simulink model "CopyModel"  (R2019b)
settings: Solver=VariableStepAuto  StartTime=0.0  StopTime=10.0  RelTol=1e-3
values from neighbouring files (symbols this model uses):
  etcModeCmd = 0    [F28379D_benchTest_CPU1.sldd]
  etcModes : value not decoded    [F28379D_benchTest_CPU1.sldd]
  etcSubModeCmd = 0    [F28379D_benchTest_CPU1.sldd]
  etcSubModes : value not decoded    [F28379D_benchTest_CPU1.sldd]
  motorControlMode = 0    [F28379D_benchTest_CPU1.sldd]
  motorPosGainI = 0.0    [F28379D_benchTest_CPU1.sldd]
  motorPosGainP = 2000.0    [F28379D_benchTest_CPU1.sldd]
  motorVelGainFeedback = 200.0    [F28379D_benchTest_CPU1.sldd]
  motorVelGainI = 2000.0    [F28379D_benchTest_CPU1.sldd]
  motorVelGainP = 200.0    [F28379D_benchTest_CPU1.sldd]
  throttlePosInputMode = 0    [F28379D_benchTest_CPU1.sldd]
  throttlePosInputModes : value not decoded    [F28379D_benchTest_CPU1.sldd]
undefined symbols (not defined in the file or in its folder): motor1PWM, motor2PWM, motorPosCommand_deg
libraries: simulink x30, c280xlib x10, canmsglib x9, FunctionCallDivider x6, hdlsllib x1
settings Model: Creator=zacha  LastModifiedBy=Nick

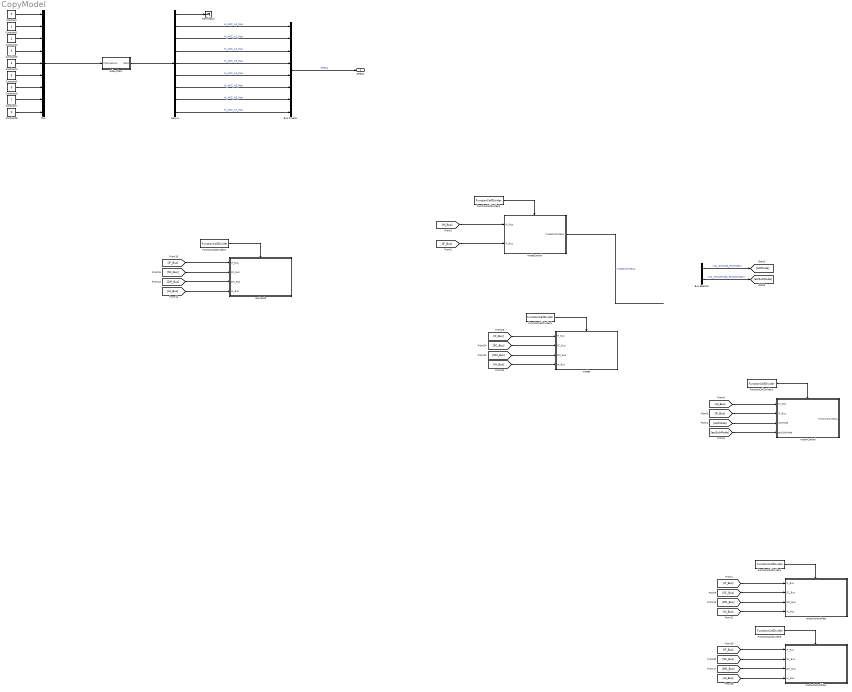
== system CopyModel ==
  Bus Creator : BusCreator  Inputs=8
  Bus Selector : BusSelector  OutputSignals=modeControlBus.SC_etcMode_etcModes,modeControlBus.SC_etcSubMode_etcSubModes
  Constant : Constant  Value=0
  Constant1 : Constant
  Constant2 : Constant  Value=2
  Constant3 : Constant  Value=3
  Constant4 : Constant  Value=4
  Constant5 : Constant  Value=5
  Constant6 : Constant  Value=6
  Constant7 : Constant  Value=7
  Constant8 : Constant  Value=0
  Demux : Demux  Outputs=9
  FunctionCallDivider1 : FunctionCallDivider/Algroithms/FunctionCallDivider  counts=1
  FunctionCallDivider2 : FunctionCallDivider/Algroithms/FunctionCallDivider  counts=10
  FunctionCallDivider3 : FunctionCallDivider/Algroithms/FunctionCallDivider  counts=10
  FunctionCallDivider4 : FunctionCallDivider/Algroithms/FunctionCallDivider  counts=1
  FunctionCallDivider5 : FunctionCallDivider/Algroithms/FunctionCallDivider  counts=100
  FunctionCallDivider6 : FunctionCallDivider/Algroithms/FunctionCallDivider  counts=10
  Mux : Mux  Inputs=9
  Subsystem : Subsystem
  Terminator : Terminator
  modeControl : Subsystem  TreatAsAtomicUnit=on
  modes : Subsystem  TreatAsAtomicUnit=on
  motorControl : Subsystem  TreatAsAtomicUnit=on
  motorControlFast : Subsystem  TreatAsAtomicUnit=on
  motorControlSlow : Subsystem  TreatAsAtomicUnit=on
  rawInputs : Subsystem  TreatAsAtomicUnit=on
  SPIBus : Outport
  wires:
  Demux/5 -> Bus Creator/4  "HI_ADC_A3_Raw"
  Bus Creator/1 -> SPIBus/1  "SPIBus"
  Constant4/1 -> Mux/5
  Mux/1 -> Subsystem/1(ChannelNum)
  Demux/7 -> Bus Creator/6  "HI_ADC_A5_Raw"
  Demux/4 -> Bus Creator/3  "HI_ADC_A2_Raw"
  Demux/2 -> Bus Creator/1  "HI_ADC_A0_Raw"
  Constant1/1 -> Mux/2
  Demux/3 -> Bus Creator/2  "HI_ADC_A1_Raw"
  Demux/8 -> Bus Creator/7  "HI_ADC_A6_Raw"
  Demux/9 -> Bus Creator/8  "HI_ADC_A7_Raw"
  Constant7/1 -> Mux/8
  Constant2/1 -> Mux/3
  Constant8/1 -> Mux/9
  Constant5/1 -> Mux/6
  Demux/6 -> Bus Creator/5  "HI_ADC_A4_Raw"
  Subsystem/1(Data) -> Demux/1
  Constant3/1 -> Mux/4
  Demux/1 -> Terminator/1
  Constant6/1 -> Mux/7
  Constant/1 -> Mux/1
  FunctionCallDivider3/1 -> rawInputs/Trigger
  [SC_Bus] -> rawInputs/2(SC_Bus)
  [IF_Bus] -> rawInputs/1(IF_Bus)
  [HI_Bus] -> rawInputs/4(HI_Bus)
  [DM_Bus] -> rawInputs/3(DM_Bus)
  [HI_Bus] -> modeControl/1(HI_Bus)
  Bus Selector/2 -> [etcSubMode]  "<SC_etcSubMode_etcSubModes>"
  modeControl/1(modeControlBus) -> ?  "modeControlBus"
  FunctionCallDivider2/1 -> modeControl/Trigger
  Bus Selector/1 -> [etcMode]  "<SC_etcMode_etcModes>"
  ? -> Bus Selector/1  "SC_Bus"
  [IF_Bus] -> modeControl/2(IF_Bus)
  [SC_Bus] -> modes/2(SC_Bus)
  FunctionCallDivider5/1 -> modes/Trigger
  [DM_Bus] -> modes/3(DM_Bus)
  [HI_Bus] -> modes/4(HI_Bus)
  [IF_Bus] -> modes/1(IF_Bus)
  FunctionCallDivider1/1 -> motorControl/Trigger
  [IF_Bus] -> motorControl/2(IF_Bus)
  [etcSubMode] -> motorControl/4(etcSubMode)
  [HI_Bus] -> motorControl/1(HI_Bus)
  [etcMode] -> motorControl/3(etcMode)
  FunctionCallDivider4/1 -> motorControlFast/Trigger
  [IF_Bus] -> motorControlSlow/1(IF_Bus)
  [DM_Bus] -> motorControlFast/3(DM_Bus)
  [SC_Bus] -> motorControlSlow/2(SC_Bus)
  [DM_Bus] -> motorControlSlow/3(DM_Bus)
  [HI_Bus] -> motorControlSlow/4(HI_Bus)
  FunctionCallDivider6/1 -> motorControlSlow/Trigger
  [HI_Bus] -> motorControlFast/4(HI_Bus)
  [IF_Bus] -> motorControlFast/1(IF_Bus)
  [SC_Bus] -> motorControlFast/2(SC_Bus)

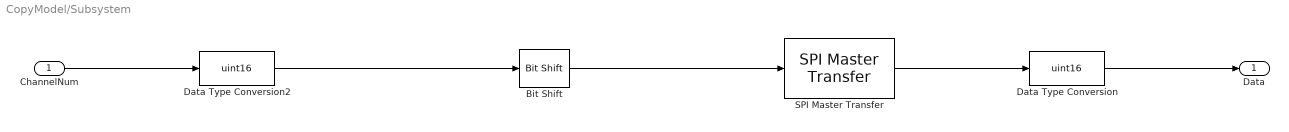
== system CopyModel/Subsystem ==
  ChannelNum : Inport
  Bit Shift : hdlsllib/Logic and Bit Operations/Bit Shift  mode=Shift Left Logical  N=11
      settings: SourceProductName=Simulink
  Data Type Conversion : DataTypeConversion  OutDataTypeStr=uint16
  Data Type Conversion2 : DataTypeConversion  OutDataTypeStr=uint16
  SPI Master Transfer : c280xlib/SPI Master Transfer  SPISelect=SPI_B  ClockPolarity=Falling_edge  ClockPhase=No_delay  SPIModule=uint32(0)  Mode=Master  BusSpeed=uint32(1000000)  FirstBitToTransfer=Most significant bit (MSB)  ClockMode=0  BlockFunction=Transfer  EnableRegisterAddress=on  RegisterAddress=0  OutputDataType=int8  OutputDataLength=1  DataBits=16  UseCustomSSPin=Explicit GPIO calls  ActiveLowSSPin=Active low  Pin=66
      settings: SourceProductName=Embedded Coder Support Package for Texas Instruments C2000 Processors  SourceProductBaseCode=TIC2000
  Data : Outport
  wires:
  ChannelNum/1 -> Data Type Conversion2/1
  Data Type Conversion/1 -> Data/1
  SPI Master Transfer/1 -> Data Type Conversion/1
  Data Type Conversion2/1 -> Bit Shift/1
  Bit Shift/1 -> SPI Master Transfer/1

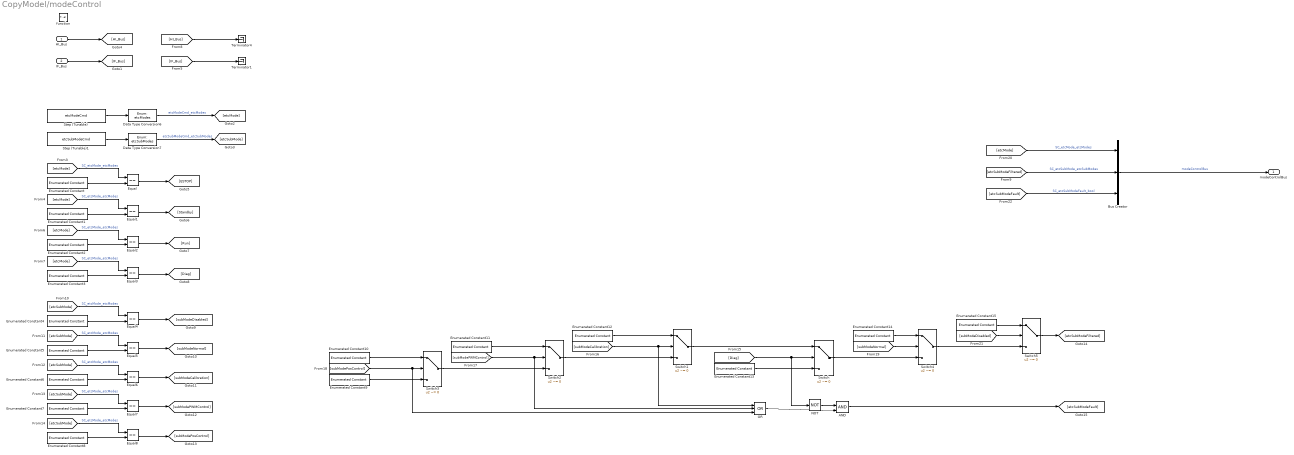
== system CopyModel/modeControl ==
  HI_Bus : Inport
  IF_Bus : Inport  Port=2
  function : TriggerPort  TriggerType=function-call  VariantControl=Variant
  AND : Logic  IconShape=distinctive  AllPortsSameDT=off  OutDataTypeStr=boolean
  Bus Creator : BusCreator  Inputs=3
  Data Type Conversion6 : DataTypeConversion  OutDataTypeStr=Enum: etcModes
  Data Type Conversion7 : DataTypeConversion  OutDataTypeStr=Enum: etcSubModes
  Enumerated Constant : simulink/Sources/Enumerated Constant  OutDataTypeStr=Enum: etcModes  Value=etcModes.ESTOP  SampleTime=inf
      settings: SourceProductName=Simulink
  Enumerated Constant1 : simulink/Sources/Enumerated Constant  OutDataTypeStr=Enum: etcModes  Value=etcModes.Standby  SampleTime=inf
      settings: SourceProductName=Simulink
  Enumerated Constant10 : simulink/Sources/Enumerated Constant  OutDataTypeStr=Enum: etcSubModes  Value=etcSubModes.PositionControl  SampleTime=inf
      settings: SourceProductName=Simulink
  Enumerated Constant11 : simulink/Sources/Enumerated Constant  OutDataTypeStr=Enum: etcSubModes  Value=etcSubModes.PWMControl  SampleTime=inf
      settings: SourceProductName=Simulink
  Enumerated Constant12 : simulink/Sources/Enumerated Constant  OutDataTypeStr=Enum: etcSubModes  Value=etcSubModes.Calibration  SampleTime=inf
      settings: SourceProductName=Simulink
  Enumerated Constant{4,9,13,15} (4 alike) : simulink/Sources/Enumerated Constant  OutDataTypeStr=Enum: etcSubModes  Value=etcSubModes.Disabled  SampleTime=inf
      settings: SourceProductName=Simulink
  Enumerated Constant14 : simulink/Sources/Enumerated Constant  OutDataTypeStr=Enum: etcSubModes  Value=etcSubModes.Normal  SampleTime=inf
      settings: SourceProductName=Simulink
  Enumerated Constant2 : simulink/Sources/Enumerated Constant  OutDataTypeStr=Enum: etcModes  Value=etcModes.Run  SampleTime=inf
      settings: SourceProductName=Simulink
  Enumerated Constant3 : simulink/Sources/Enumerated Constant  OutDataTypeStr=Enum: etcModes  Value=etcModes.Diag  SampleTime=inf
      settings: SourceProductName=Simulink
  Enumerated Constant5 : simulink/Sources/Enumerated Constant  OutDataTypeStr=Enum: etcSubModes  Value=etcSubModes.Normal  SampleTime=inf
      settings: SourceProductName=Simulink
  Enumerated Constant6 : simulink/Sources/Enumerated Constant  OutDataTypeStr=Enum: etcSubModes  Value=etcSubModes.Calibration  SampleTime=inf
      settings: SourceProductName=Simulink
  Enumerated Constant7 : simulink/Sources/Enumerated Constant  OutDataTypeStr=Enum: etcSubModes  Value=etcSubModes.PWMControl  SampleTime=inf
      settings: SourceProductName=Simulink
  Enumerated Constant8 : simulink/Sources/Enumerated Constant  OutDataTypeStr=Enum: etcSubModes  Value=etcSubModes.PositionControl  SampleTime=inf
      settings: SourceProductName=Simulink
  Equal{,1..8} (9 alike) : RelationalOperator  Operator===  OutDataTypeStr=boolean  RndMeth=Simplest
  NOT : Logic  Operator=NOT  IconShape=distinctive  AllPortsSameDT=off  OutDataTypeStr=boolean
  OR : Logic  Operator=OR  Inputs=3  IconShape=distinctive  AllPortsSameDT=off  OutDataTypeStr=boolean
  Step (Tunable) : Constant  Value=etcModeCmd  VectorParams1D=off  SampleTime=-1
  Step (Tunable)1 : Constant  Value=etcSubModeCmd  VectorParams1D=off  SampleTime=-1
  Switch{,1..5} (6 alike) : Switch  Criteria=u2 ~= 0
  Terminator1 : Terminator
  Terminator4 : Terminator
  modeControlBus : Outport
  wires:
  IF_Bus/1 -> [IF_Bus]
  [HI_Bus] -> Terminator4/1
  HI_Bus/1 -> [HI_Bus]
  [IF_Bus] -> Terminator1/1
  Bus Creator/1 -> modeControlBus/1  "modeControlBus"
  [etcMode] -> Bus Creator/1  "SC_etcMode_etcModes"
  [etcMode] -> Equal/1  "SC_etcMode_etcModes"
  Enumerated Constant/1 -> Equal/2
  Equal/1 -> [ESTOP]
  Equal1/1 -> [Standby]
  [etcMode] -> Equal1/1  "SC_etcMode_etcModes"
  Enumerated Constant1/1 -> Equal1/2
  Equal2/1 -> [Run]
  Enumerated Constant2/1 -> Equal2/2
  [etcMode] -> Equal2/1  "SC_etcMode_etcModes"
  Enumerated Constant3/1 -> Equal3/2
  [etcMode] -> Equal3/1  "SC_etcMode_etcModes"
  Equal3/1 -> [Diag]
  [etcSubModeFiltered] -> Bus Creator/2  "SC_etcSubMode_etcSubModes"
  Equal4/1 -> [subModeDisabled]
  [etcSubMode] -> Equal4/1  "SC_etcMode_etcModes"
  Enumerated Constant4/1 -> Equal4/2
  Enumerated Constant5/1 -> Equal5/2
  Equal5/1 -> [subModeNormal]
  [etcSubMode] -> Equal5/1  "SC_etcMode_etcModes"
  Enumerated Constant6/1 -> Equal6/2
  Equal6/1 -> [subModeCalibration]
  [etcSubMode] -> Equal6/1  "SC_etcMode_etcModes"
  Enumerated Constant7/1 -> Equal7/2
  Equal7/1 -> [subModePWMControl]
  [etcSubMode] -> Equal7/1  "SC_etcMode_etcModes"
  Enumerated Constant8/1 -> Equal8/2
  Equal8/1 -> [subModePosControl]
  [etcSubMode] -> Equal8/1  "SC_etcMode_etcModes"
  [Diag] -> NOT/1, Switch/2
  Switch1/1 -> Switch/1
  [subModeCalibration] -> OR/1, Switch1/2
  [subModePWMControl] -> OR/2, Switch2/2
  Switch2/1 -> Switch1/3
  [subModePosControl] -> OR/3, Switch3/2
  Switch3/1 -> Switch2/3
  Enumerated Constant9/1 -> Switch3/3
  Enumerated Constant10/1 -> Switch3/1
  Enumerated Constant11/1 -> Switch2/1
  Enumerated Constant12/1 -> Switch1/1
  Enumerated Constant13/1 -> Switch/3
  Switch/1 -> Switch4/3
  [subModeNormal] -> Switch4/2
  Enumerated Constant14/1 -> Switch4/1
  Enumerated Constant15/1 -> Switch5/1
  Switch4/1 -> Switch5/3
  [subModeDisabled] -> Switch5/2
  Switch5/1 -> [etcSubModeFiltered]
  OR/1 -> AND/2
  AND/1 -> [etcSubModeFault]
  [etcSubModeFault] -> Bus Creator/3  "SC_etcSubModeFault_bool"
  NOT/1 -> AND/1
  Step (Tunable)1/1 -> Data Type Conversion7/1
  Data Type Conversion7/1 -> [etcSubMode]  "etcSubModeCmd_etcSubModes"
  Step (Tunable)/1 -> Data Type Conversion6/1
  Data Type Conversion6/1 -> [etcMode]  "etcModeCmd_etcModes"

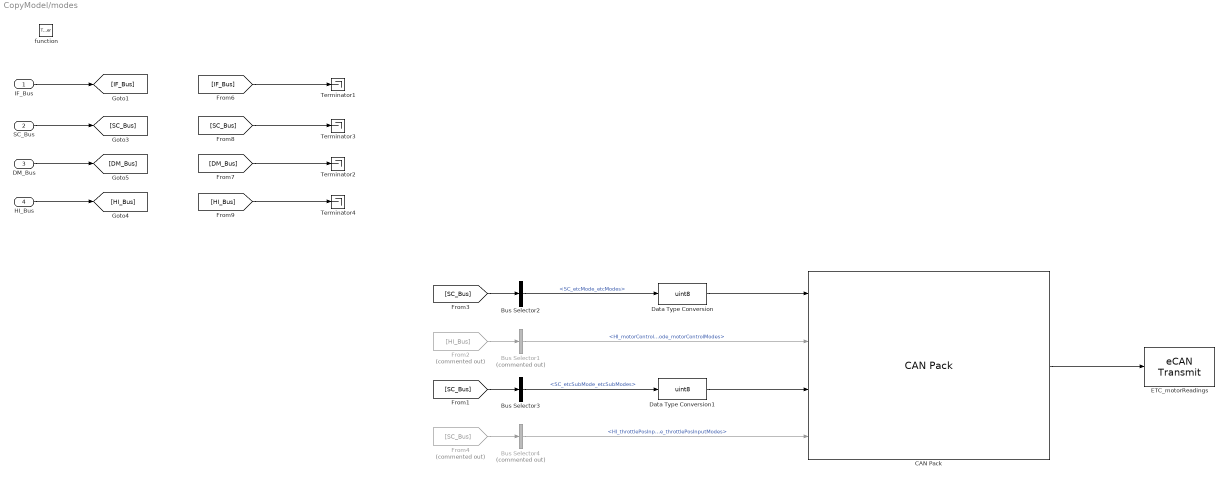
== system CopyModel/modes ==
  IF_Bus : Inport
  SC_Bus : Inport  Port=2
  DM_Bus : Inport  Port=3
  HI_Bus : Inport  Port=4
  function : TriggerPort  TriggerType=function-call  VariantControl=Variant
  Bus Selector1 : BusSelector  Commented=on  OutputSignals=VectorBoxBus.HI_motorControlMode_motorControlModes
  Bus Selector2 : BusSelector  OutputSignals=modeControlBus.SC_etcMode_etcModes
  Bus Selector3 : BusSelector  OutputSignals=modeControlBus.SC_etcSubMode_etcSubModes
  Bus Selector4 : BusSelector  Commented=on  OutputSignals=VectorBoxBus.HI_throttlePosInputMode_throttlePosInputModes
  CAN Pack : canmsglib/CAN Pack  CANdbFile=C:\Git\ETC-Development\DBCs\F28377S_etc_benchTest.dbc  MsgList=ETC_modes  MsgName=ETC_modes  MsgIDType=Standard (11-bit identifier)  MsgIdentifier=1000  MsgLength=4  Remote=off  ApplyMinMax=off  BusOutput=off  SignalInfo={'ETC_mode','0','8','LE','unsigned','Standard','0','1','0','0','255';'ETC_motorControlMode','16','8','LE','unsigned','Standard','0','1','0','0','255';'ETC_subMode','8','8','LE','unsigned','Standard','0','1','0','0','255';'ETC_throttlePosInputMode','24','8','LE','unsigned','Standard','0','1','0','0','255'}
      settings: SourceProductName=Vehicle Network Toolbox  SourceProductBaseCode=VN  DataFormat=CANdb specified signals
  Data Type Conversion : DataTypeConversion  OutDataTypeStr=uint8
  Data Type Conversion1 : DataTypeConversion  OutDataTypeStr=uint8
  ETC_motorReadings : c280xlib/eCAN Transmit  chipFamily=C280x  useModule=eCAN_A  mailboxNo=13  messageID=0  messageType=Standard (11-bit identifier)  enableBlockingMode=off  postInterrupt=off  interruptLine=0
      settings: SourceProductName=Embedded Coder Support Package for Texas Instruments C2000 Processors  SourceProductBaseCode=TIC2000
  From2 : From  Commented=on  GotoTag=HI_Bus
  From4 : From  Commented=on  GotoTag=SC_Bus
  Terminator{1..4} (4 alike) : Terminator
  wires:
  From4/1 -> Bus Selector4/1
  Bus Selector4/1 -> CAN Pack/4  "<HI_throttlePosInputMode_throttlePosInputModes>"
  [SC_Bus] -> Bus Selector3/1
  Bus Selector3/1 -> Data Type Conversion1/1  "<SC_etcSubMode_etcSubModes>"
  IF_Bus/1 -> [IF_Bus]
  [HI_Bus] -> Terminator4/1
  HI_Bus/1 -> [HI_Bus]
  SC_Bus/1 -> [SC_Bus]
  DM_Bus/1 -> [DM_Bus]
  [SC_Bus] -> Terminator3/1
  [DM_Bus] -> Terminator2/1
  [IF_Bus] -> Terminator1/1
  Bus Selector1/1 -> CAN Pack/2  "<HI_motorControlMode_motorControlModes>"
  Bus Selector2/1 -> Data Type Conversion/1  "<SC_etcMode_etcModes>"
  From2/1 -> Bus Selector1/1
  [SC_Bus] -> Bus Selector2/1
  CAN Pack/1 -> ETC_motorReadings/1
  Data Type Conversion/1 -> CAN Pack/1
  Data Type Conversion1/1 -> CAN Pack/3

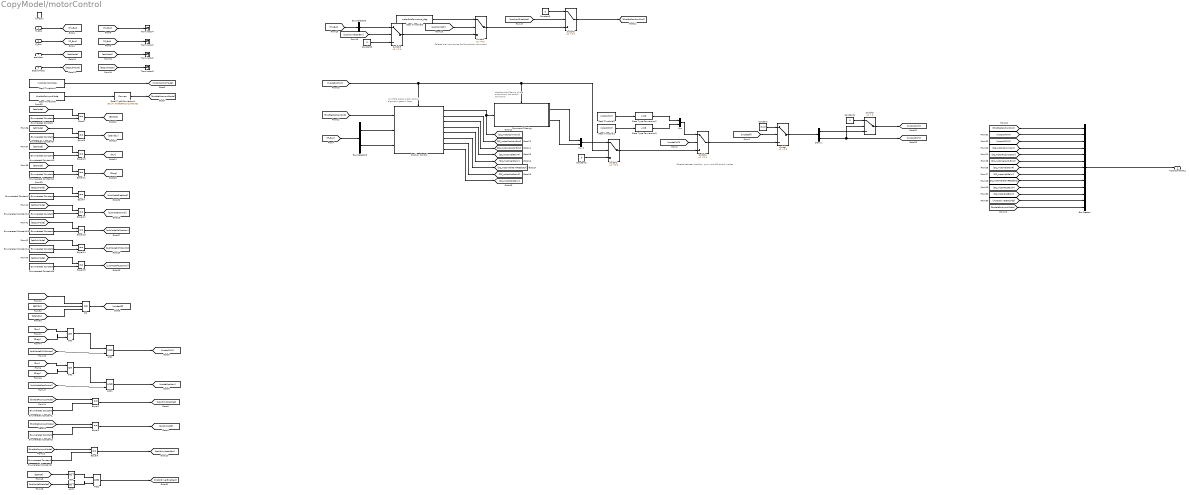
== system CopyModel/motorControl ==
  note: Selects the input source for the position command
  note: Selects between position, pwm, and off control modes
  note: Handles the filtering of the output from the control command
  note: All of the actual motor control algorithm goes in here
  HI_Bus : Inport
  IF_Bus : Inport  Port=2
  etcMode : Inport  Port=3
  etcSubMode : Inport  Port=4
  function : TriggerPort  TriggerType=function-call  VariantControl=Variant
  AND : Logic  IconShape=distinctive  AllPortsSameDT=off  OutDataTypeStr=boolean
  AND1 : Logic  IconShape=distinctive  AllPortsSameDT=off  OutDataTypeStr=boolean
  AND2 : Logic  IconShape=distinctive  AllPortsSameDT=off  OutDataTypeStr=boolean
  Bus Creator : BusCreator  Inputs=13
  Bus Selector3 : BusSelector  OutputSignals=AnalogInputFiltering_Bus.ExternalADCBus.IF_throttlePos1_pct,AnalogInputFiltering_Bus.ExternalADCBus.IF_throttleVel1_degS
  Bus Selector6 : BusSelector  OutputSignals=VectorBoxBus.HI_throttleCmd_pct
  Command Filtering : Subsystem
  Constant : Constant  Value=[0 0]
  Constant{1..4} (4 alike) : Constant  Value=0
  Data Type Conversion1 : DataTypeConversion  OutDataTypeStr=Enum: throttlePosInputModes
  Data Type Conversion2 : DataTypeConversion  OutDataTypeStr=uint8
  Data Type Conversion3 : DataTypeConversion  OutDataTypeStr=uint8
  Demux : Demux  Outputs=2
  Enumerated Constant : simulink/Sources/Enumerated Constant  OutDataTypeStr=Enum: etcModes  Value=etcModes.ESTOP  SampleTime=inf
      settings: SourceProductName=Simulink
  Enumerated Constant1 : simulink/Sources/Enumerated Constant  OutDataTypeStr=Enum: throttlePosInputModes  Value=throttlePosInputModes.Disabled  SampleTime=inf
      settings: SourceProductName=Simulink
  Enumerated Constant10 : simulink/Sources/Enumerated Constant  OutDataTypeStr=Enum: etcModes  Value=etcModes.Run  SampleTime=inf
      settings: SourceProductName=Simulink
  Enumerated Constant11 : simulink/Sources/Enumerated Constant  OutDataTypeStr=Enum: etcModes  Value=etcModes.Diag  SampleTime=inf
      settings: SourceProductName=Simulink
  Enumerated Constant12 : simulink/Sources/Enumerated Constant  OutDataTypeStr=Enum: etcSubModes  Value=etcSubModes.Normal  SampleTime=inf
      settings: SourceProductName=Simulink
  Enumerated Constant13 : simulink/Sources/Enumerated Constant  OutDataTypeStr=Enum: etcSubModes  Value=etcSubModes.Calibration  SampleTime=inf
      settings: SourceProductName=Simulink
  Enumerated Constant14 : simulink/Sources/Enumerated Constant  OutDataTypeStr=Enum: etcSubModes  Value=etcSubModes.PWMControl  SampleTime=inf
      settings: SourceProductName=Simulink
  Enumerated Constant15 : simulink/Sources/Enumerated Constant  OutDataTypeStr=Enum: etcSubModes  Value=etcSubModes.PositionControl  SampleTime=inf
      settings: SourceProductName=Simulink
  Enumerated Constant3 : simulink/Sources/Enumerated Constant  OutDataTypeStr=Enum: throttlePosInputModes  Value=throttlePosInputModes.CCP  SampleTime=inf
      settings: SourceProductName=Simulink
  Enumerated Constant6 : simulink/Sources/Enumerated Constant  OutDataTypeStr=Enum: throttlePosInputModes  Value=throttlePosInputModes.VectorBox  SampleTime=inf
      settings: SourceProductName=Simulink
  Enumerated Constant7 : simulink/Sources/Enumerated Constant  OutDataTypeStr=Enum: etcSubModes  Value=etcSubModes.Disabled  SampleTime=inf
      settings: SourceProductName=Simulink
  Enumerated Constant9 : simulink/Sources/Enumerated Constant  OutDataTypeStr=Enum: etcModes  Value=etcModes.Standby  SampleTime=inf
      settings: SourceProductName=Simulink
  Equal{,1,3,6..7,9..15} (12 alike) : RelationalOperator  Operator===  OutDataTypeStr=boolean  RndMeth=Simplest
  Mux : Mux  Inputs=2
  Mux1 : Mux  Inputs=2
  NOT : Logic  Operator=NOT  IconShape=distinctive  AllPortsSameDT=off  OutDataTypeStr=boolean
  NOT1 : Logic  Operator=NOT  IconShape=distinctive  AllPortsSameDT=off  OutDataTypeStr=boolean
  OR : Logic  Operator=OR  Inputs=3  IconShape=distinctive  AllPortsSameDT=off  OutDataTypeStr=boolean
  OR1 : Logic  Operator=OR  IconShape=distinctive  AllPortsSameDT=off  OutDataTypeStr=boolean
  OR2 : Logic  Operator=OR  IconShape=distinctive  AllPortsSameDT=off  OutDataTypeStr=boolean
  Position Control : Subsystem  TreatAsAtomicUnit=on
  Step (Tunable)1 : Constant  Value=motor2PWM  VectorParams1D=off  SampleTime=-1
  Step (Tunable)2 : Constant  Value=motor1PWM  VectorParams1D=off  SampleTime=-1
  Step (Tunable)4 : Constant  Value=motorControlMode  VectorParams1D=off  SampleTime=-1
  Step (Tunable)5 : Constant  Value=motorPosCommand_deg  VectorParams1D=off  SampleTime=-1
  Step (Tunable)6 : Constant  Value=throttlePosInputMode  VectorParams1D=off  SampleTime=-1
  Switch{,1..5} (6 alike) : Switch  Criteria=u2 ~= 0
  Switch6 : Switch  Criteria=u2 > Threshold
  Terminator{1..4} (4 alike) : Terminator
  motorControlBus : Outport
  wires:
  IF_Bus/1 -> [IF_Bus]
  [HI_Bus] -> Terminator4/1
  HI_Bus/1 -> [HI_Bus]
  [IF_Bus] -> Terminator1/1
  Bus Creator/1 -> motorControlBus/1  "motorControlBus"
  Switch/1 -> Demux/1
  Demux/1 -> Switch6/3  "SC_motor1PWM_pct"
  Demux/2 -> [motor2PWM], Switch6/2  "SC_motor2PWM_pct"
  [modeOff] -> Switch/2
  Constant/1 -> Switch/1
  Switch1/1 -> Switch/3
  [modePWM] -> Switch1/2
  Mux/1 -> Switch1/1
  Mux1/1 -> Switch2/1
  Switch2/1 -> Switch1/3
  Constant1/1 -> Switch2/3
  [IF_Bus] -> Bus Selector3/1
  [modePosition] -> Command Filtering/Enable, Switch2/2, Position Control/Enable
  Position Control/1(velCmd) -> [SC_motorCommand], Command Filtering/1(SC_motorCommand)  "SC_motorCommand"
  Bus Selector3/2 -> Position Control/3(throttleVelIn)  "<IF_throttleVel1_degS>"
  Bus Selector3/1 -> Position Control/2(throttlePos)  "<IF_throttlePos1_pct>"
  Command Filtering/1(SC_motor1PWM_pct) -> Mux1/1
  Command Filtering/2(SC_motor2PWM_pct) -> Mux1/2
  AND1/1 -> [modePosition]
  AND/1 -> [modePWM]
  [subModeDisabled] -> OR/1
  Switch3/1 -> Switch4/3
  Switch4/1 -> Switch5/3
  Data Type Conversion1/1 -> [throttlePosInputMode]
  Equal1/1 -> [positionDisabled]
  Enumerated Constant1/1 -> Equal1/2
  [throttlePosInputMode] -> Equal1/1
  Equal3/1 -> [positionCCP]
  Enumerated Constant3/1 -> Equal3/2
  [throttlePosInputMode] -> Equal3/1
  Equal6/1 -> [positionVectorBox]
  Enumerated Constant6/1 -> Equal6/2
  [throttlePosInputMode] -> Equal6/1
  Constant2/1 -> Switch3/3
  Constant3/1 -> Switch5/1
  [positionDisabled] -> Switch5/2
  [positionCCP] -> Switch4/2
  [positionVectorBox] -> Switch3/2
  Bus Selector6/1 -> Switch3/1  "<HI_throttleCmd_pct>"
  [HI_Bus] -> Bus Selector6/1
  Switch5/1 -> [throttlePositionCmd]
  [throttlePositionCmd] -> Position Control/1(motorPosCmd)
  [throttlePositionCmd] -> Bus Creator/1  "SC_throttlePositionCmd_pct"
  Position Control/2(motorPosError) -> [SC_motorPositionError]  "SC_motorPositionError"
  Position Control/3(motorVelError) -> [SC_motorVelocityError]  "SC_motorVelocityError"
  [SC_motorVelocityError] -> Bus Creator/6  "SC_motorVelocityError"
  [SC_motorPositionError] -> Bus Creator/5  "SC_motorPositionError"
  [SC_motorCommand] -> Bus Creator/4  "SC_motorCommand"
  Position Control/4(motorVelGainP) -> [SC_motorVelGainP]  "SC_motorVelGainP"
  Position Control/5(motorVelGainI) -> [SC_motorVelGainI]  "SC_motorVelGainI"
  Position Control/6(motorVelGainFeedback) -> [SC_motorVelGainFeedback]  "SC_motorVelGainFeedback"
  Position Control/7(motorPosGainP) -> [SC_motorPosGainP]  "SC_motorPosGainP"
  Position Control/8(motorPosGainI) -> [SC_motorPosGainI]  "SC_motorPosGainI"
  [SC_motorPosGainI] -> Bus Creator/11  "SC_motorPosGainI"
  [SC_motorPosGainP] -> Bus Creator/10  "SC_motorPosGainP"
  [SC_motorVelGainFeedback] -> Bus Creator/9  "SC_motorVelGainFeedback"
  [SC_motorVelGainI] -> Bus Creator/8  "SC_motorVelGainI"
  [SC_motorVelGainP] -> Bus Creator/7  "SC_motorVelGainP"
  etcMode/1 -> [etcMode]
  [etcMode] -> Terminator2/1
  OR/1 -> [modeOff]
  [ESTOP] -> OR/2
  [Standby] -> OR/3
  etcSubMode/1 -> [etcSubMode]
  [etcSubMode] -> Terminator3/1
  Equal9/1 -> [Standby]
  Enumerated Constant9/1 -> Equal9/2
  [etcMode] -> Equal10/1  "SC_etcMode_etcModes"
  Equal/1 -> [ESTOP]
  [etcMode] -> Equal9/1  "SC_etcMode_etcModes"
  Equal10/1 -> [Run]
  Equal11/1 -> [Diag]
  [etcMode] -> Equal11/1  "SC_etcMode_etcModes"
  [etcMode] -> Equal/1  "SC_etcMode_etcModes"
  Enumerated Constant/1 -> Equal/2
  Enumerated Constant11/1 -> Equal11/2
  Enumerated Constant10/1 -> Equal10/2
  Enumerated Constant7/1 -> Equal7/2
  Equal7/1 -> [subModeDisabled]
  [etcSubMode] -> Equal7/1  "SC_etcMode_etcModes"
  Equal13/1 -> [subModeCalibration]
  [etcSubMode] -> Equal13/1  "SC_etcMode_etcModes"
  Enumerated Constant13/1 -> Equal13/2
  Enumerated Constant14/1 -> Equal14/2
  [etcSubMode] -> Equal12/1  "SC_etcMode_etcModes"
  Equal15/1 -> [subModePosControl]
  Equal14/1 -> [subModePWMControl]
  Enumerated Constant12/1 -> Equal12/2
  Equal12/1 -> [subModeNormal]
  Enumerated Constant15/1 -> Equal15/2
  [etcSubMode] -> Equal15/1  "SC_etcMode_etcModes"
  [etcSubMode] -> Equal14/1  "SC_etcMode_etcModes"
  [Run] -> OR1/1
  [Diag] -> OR1/2
  OR1/1 -> AND/1
  [subModePWMControl] -> AND/2
  OR2/1 -> AND1/1
  [subModePosControl] -> AND1/2
  [Run] -> OR2/1
  [Diag] -> OR2/2
  [ESTOP] -> NOT/1
  [subModeDisabled] -> NOT1/1
  NOT/1 -> AND2/1
  NOT1/1 -> AND2/2
  AND2/1 -> [motorDriverEnabled]
  [motorDriverEnabled] -> Bus Creator/12  "SC_motorDriverEnabled_bool"
  [motor1PWM] -> Bus Creator/2  "SC_motor1PWM_pct"
  [motor2PWM] -> Bus Creator/3  "SC_motor2PWM_pct"
  Constant4/1 -> Switch6/1
  Switch6/1 -> [motor1PWM]  "SC_motor1PWM_pct"
  Step (Tunable)6/1 -> Data Type Conversion1/1  "throttlePosInputMode_throttlePosInputModes"
  [throttlePosInputMode] -> Bus Creator/13  "SC_throttlePosInputMode_throttlePosInputModes"
  Step (Tunable)4/1 -> [motorControlMode]  "motorControlMode_motorControlModes"
  Step (Tunable)5/1 -> Switch4/1  "motorPosCmd_deg"
  Step (Tunable)1/1 -> Data Type Conversion3/1  "motor2PWM_pct"
  Data Type Conversion3/1 -> Mux/2  "motor2PWM_pct"
  Data Type Conversion2/1 -> Mux/1  "motor1PWM_pct"
  Step (Tunable)2/1 -> Data Type Conversion2/1  "motor1PWM_pct"

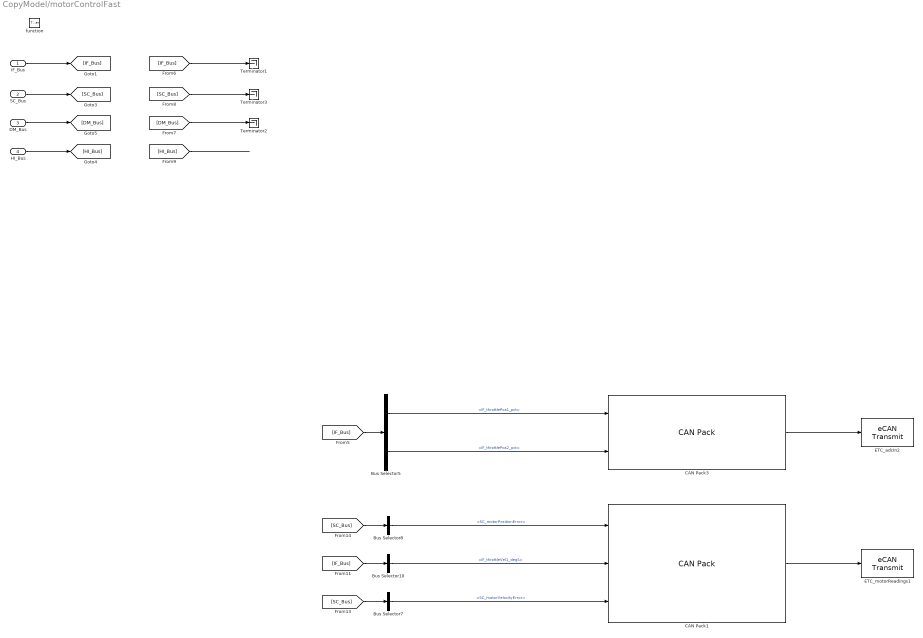
== system CopyModel/motorControlFast ==
  IF_Bus : Inport
  SC_Bus : Inport  Port=2
  DM_Bus : Inport  Port=3
  HI_Bus : Inport  Port=4
  function : TriggerPort  TriggerType=function-call  VariantControl=Variant
  Bus Selector10 : BusSelector  OutputSignals=AnalogInputFiltering_Bus.ExternalADCBus.IF_throttleVel1_degS
  Bus Selector5 : BusSelector  OutputSignals=AnalogInputFiltering_Bus.ExternalADCBus.IF_throttlePos1_pct,AnalogInputFiltering_Bus.ExternalADCBus.IF_throttlePos2_pct
  Bus Selector7 : BusSelector  OutputSignals=motorControlBus.SC_motorVelocityError
  Bus Selector8 : BusSelector  OutputSignals=motorControlBus.SC_motorPositionError
  CAN Pack1 : canmsglib/CAN Pack  CANdbFile=C:\Git\ETC-Development\DBCs\F28377S_etc_benchTest.dbc  MsgList=ETC_adcRaw1  MsgName=ETC_motorControlData1  MsgIDType=Standard (11-bit identifier)  MsgIdentifier=1002  MsgLength=6  Remote=off  ApplyMinMax=off  BusOutput=off  SignalInfo={ 'ETC_motorPositionError', '0', '16', 'LE', 'signed', 'Standard', '0', '0.01', '0', '-327.68', '327.67'; 'ETC_motorVelocity', '16', '16', 'LE', 'signed', 'Standard', '0', '0.01', '0', '-327.68', '327.67'; 'ETC_motorVelocityError', '32', '16', 'LE', 'signed', 'Standard', '0', '0.01', '0', '-327.68', '327.67' }
      settings: SourceProductName=Vehicle Network Toolbox  SourceProductBaseCode=VN  DataFormat=CANdb specified signals
  CAN Pack3 : canmsglib/CAN Pack  CANdbFile=C:\Git\ETC-Development\DBCs\F28377S_etc_benchTest.dbc  MsgList=ETC_adcRaw1  MsgName=ETC_throttlePosition  MsgIDType=Standard (11-bit identifier)  MsgIdentifier=1010  MsgLength=4  Remote=off  ApplyMinMax=off  BusOutput=off  SignalInfo={ 'ETC_throttlePosition1', '0', '16', 'LE', 'unsigned', 'Standard', '0', '0.01', '0', '0', '655.35'; 'ETC_throttlePosition2', '16', '16', 'LE', 'unsigned', 'Standard', '0', '0.01', '0', '0', '655.35' }
      settings: SourceProductName=Vehicle Network Toolbox  SourceProductBaseCode=VN  DataFormat=CANdb specified signals
  ETC_adcIn2 : c280xlib/eCAN Transmit  chipFamily=C280x  useModule=eCAN_A  mailboxNo=7  messageID=0  messageType=Standard (11-bit identifier)  enableBlockingMode=off  postInterrupt=off  interruptLine=0
      settings: SourceProductName=Embedded Coder Support Package for Texas Instruments C2000 Processors  SourceProductBaseCode=TIC2000
  ETC_motorReadings1 : c280xlib/eCAN Transmit  chipFamily=C280x  useModule=eCAN_A  mailboxNo=10  messageID=0  messageType=Standard (11-bit identifier)  enableBlockingMode=off  postInterrupt=off  interruptLine=0
      settings: SourceProductName=Embedded Coder Support Package for Texas Instruments C2000 Processors  SourceProductBaseCode=TIC2000
  Terminator1 : Terminator
  Terminator2 : Terminator
  Terminator3 : Terminator
  wires:
  [SC_Bus] -> Bus Selector7/1
  Bus Selector8/1 -> CAN Pack1/1  "<SC_motorPositionError>"
  Bus Selector10/1 -> CAN Pack1/2  "<IF_throttleVel1_degS>"
  [IF_Bus] -> Bus Selector10/1
  [SC_Bus] -> Bus Selector8/1
  CAN Pack1/1 -> ETC_motorReadings1/1
  Bus Selector7/1 -> CAN Pack1/3  "<SC_motorVelocityError>"
  IF_Bus/1 -> [IF_Bus]
  [HI_Bus] -> ?
  HI_Bus/1 -> [HI_Bus]
  SC_Bus/1 -> [SC_Bus]
  DM_Bus/1 -> [DM_Bus]
  [SC_Bus] -> Terminator3/1
  [DM_Bus] -> Terminator2/1
  [IF_Bus] -> Terminator1/1
  Bus Selector5/1 -> CAN Pack3/1  "<IF_throttlePos1_pct>"
  CAN Pack3/1 -> ETC_adcIn2/1
  [IF_Bus] -> Bus Selector5/1
  Bus Selector5/2 -> CAN Pack3/2  "<IF_throttlePos2_pct>"

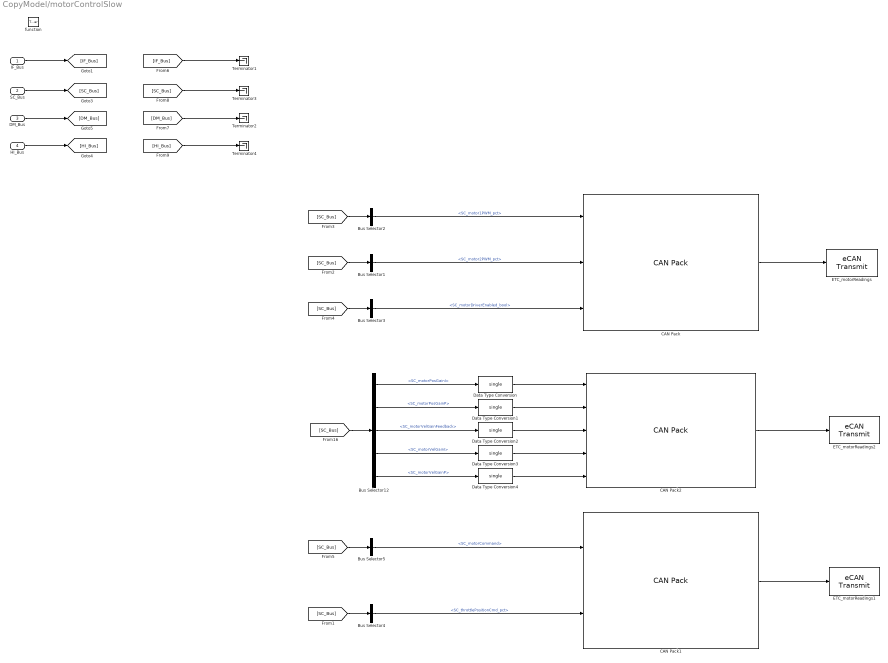
== system CopyModel/motorControlSlow ==
  IF_Bus : Inport
  SC_Bus : Inport  Port=2
  DM_Bus : Inport  Port=3
  HI_Bus : Inport  Port=4
  function : TriggerPort  TriggerType=function-call  VariantControl=Variant
  Bus Selector1 : BusSelector  OutputSignals=motorControlBus.SC_motor2PWM_pct
  Bus Selector12 : BusSelector  OutputSignals=motorControlBus.SC_motorPosGainI,motorControlBus.SC_motorPosGainP,motorControlBus.SC_motorVelGainFeedback,motorControlBus.SC_motorVelGainI,motorControlBus.SC_motorVelGainP
  Bus Selector2 : BusSelector  OutputSignals=motorControlBus.SC_motor1PWM_pct
  Bus Selector3 : BusSelector  OutputSignals=motorControlBus.SC_motorDriverEnabled_bool
  Bus Selector4 : BusSelector  OutputSignals=motorControlBus.SC_throttlePositionCmd_pct
  Bus Selector5 : BusSelector  OutputSignals=motorControlBus.SC_motorCommand
  CAN Pack : canmsglib/CAN Pack  CANdbFile=C:\Git\ETC-Development\DBCs\F28377S_etc_benchTest.dbc  MsgList=ETC_motorControl  MsgName=ETC_motorControl  MsgIDType=Standard (11-bit identifier)  MsgIdentifier=1001  MsgLength=8  Remote=off  ApplyMinMax=off  BusOutput=off  SignalInfo={'ETC_motor1PWM','0','8','LE','unsigned','Standard','0','1','0','0','255';'ETC_motor2PWM','8','8','LE','unsigned','Standard','0','1','0','0','255';'ETC_motorEnable','16','1','LE','unsigned','Standard','0','1','0','0','1'}
      settings: SourceProductName=Vehicle Network Toolbox  SourceProductBaseCode=VN  DataFormat=CANdb specified signals
  CAN Pack1 : canmsglib/CAN Pack  CANdbFile=C:\Git\ETC-Development\DBCs\F28377S_etc_benchTest.dbc  MsgList=ETC_motorControlData2  MsgName=ETC_motorControlData2  MsgIDType=Standard (11-bit identifier)  MsgIdentifier=1003  MsgLength=4  Remote=off  ApplyMinMax=off  BusOutput=off  SignalInfo={'ETC_motorCommand','16','16','LE','signed','Standard','0','1','0','-32768','32767';'ETC_throttlePositionCmd','0','16','LE','unsigned','Standard','0','0.01','0','0','655.35'}
      settings: SourceProductName=Vehicle Network Toolbox  SourceProductBaseCode=VN  DataFormat=CANdb specified signals
  CAN Pack2 : canmsglib/CAN Pack  CANdbFile=C:\Git\ETC-Development\DBCs\F28377S_etc_benchTest.dbc  MsgList=ETC_motorControlGains  MsgName=ETC_motorControlGains  MsgIDType=Standard (11-bit identifier)  MsgIdentifier=1005  MsgLength=5  Remote=off  ApplyMinMax=off  BusOutput=off  SignalInfo={'ETC_motorPosGainI','32','8','LE','unsigned','Standard','0','0.1','0','0','25.5';'ETC_motorPosGainP','24','8','LE','unsigned','Standard','0','0.1','0','0','25.5';'ETC_motorVelGainFeedback','16','8','LE','unsigned','Standard','0','0.1','0','0','25.5';'ETC_motorVelGainI','8','8','LE','unsigned','Standard','0','0.1','0','0','25.5';'ETC_motorVelGainP','0','8','LE','unsigned','Standard','0','0.1','0','0','25.5'}
      settings: SourceProductName=Vehicle Network Toolbox  SourceProductBaseCode=VN  DataFormat=CANdb specified signals
  Data Type Conversion{,1..4} (5 alike) : DataTypeConversion  OutDataTypeStr=single
  ETC_motorReadings : c280xlib/eCAN Transmit  chipFamily=C280x  useModule=eCAN_A  mailboxNo=4  messageID=0  messageType=Standard (11-bit identifier)  enableBlockingMode=off  postInterrupt=off  interruptLine=0
      settings: SourceProductName=Embedded Coder Support Package for Texas Instruments C2000 Processors  SourceProductBaseCode=TIC2000
  ETC_motorReadings1 : c280xlib/eCAN Transmit  chipFamily=C280x  useModule=eCAN_A  mailboxNo=14  messageID=0  messageType=Standard (11-bit identifier)  enableBlockingMode=off  postInterrupt=off  interruptLine=0
      settings: SourceProductName=Embedded Coder Support Package for Texas Instruments C2000 Processors  SourceProductBaseCode=TIC2000
  ETC_motorReadings2 : c280xlib/eCAN Transmit  chipFamily=C280x  useModule=eCAN_A  mailboxNo=12  messageID=0  messageType=Standard (11-bit identifier)  enableBlockingMode=off  postInterrupt=off  interruptLine=0
      settings: SourceProductName=Embedded Coder Support Package for Texas Instruments C2000 Processors  SourceProductBaseCode=TIC2000
  Terminator{1..4} (4 alike) : Terminator
  wires:
  IF_Bus/1 -> [IF_Bus]
  [HI_Bus] -> Terminator4/1
  HI_Bus/1 -> [HI_Bus]
  SC_Bus/1 -> [SC_Bus]
  DM_Bus/1 -> [DM_Bus]
  [SC_Bus] -> Terminator3/1
  [DM_Bus] -> Terminator2/1
  [IF_Bus] -> Terminator1/1
  Bus Selector3/1 -> CAN Pack/3  "<SC_motorDriverEnabled_bool>"
  Bus Selector1/1 -> CAN Pack/2  "<SC_motor2PWM_pct>"
  Bus Selector2/1 -> CAN Pack/1  "<SC_motor1PWM_pct>"
  [SC_Bus] -> Bus Selector1/1
  [SC_Bus] -> Bus Selector3/1
  [SC_Bus] -> Bus Selector2/1
  CAN Pack/1 -> ETC_motorReadings/1
  [SC_Bus] -> Bus Selector12/1
  CAN Pack2/1 -> ETC_motorReadings2/1
  Bus Selector12/1 -> Data Type Conversion/1  "<SC_motorPosGainI>"
  Bus Selector12/2 -> Data Type Conversion1/1  "<SC_motorPosGainP>"
  Bus Selector12/3 -> Data Type Conversion2/1  "<SC_motorVelGainFeedback>"
  Bus Selector12/4 -> Data Type Conversion3/1  "<SC_motorVelGainI>"
  Bus Selector12/5 -> Data Type Conversion4/1  "<SC_motorVelGainP>"
  Data Type Conversion/1 -> CAN Pack2/1
  Data Type Conversion2/1 -> CAN Pack2/3
  Data Type Conversion3/1 -> CAN Pack2/4
  Data Type Conversion4/1 -> CAN Pack2/5
  Data Type Conversion1/1 -> CAN Pack2/2
  [SC_Bus] -> Bus Selector5/1
  [SC_Bus] -> Bus Selector4/1
  Bus Selector4/1 -> CAN Pack1/2  "<SC_throttlePositionCmd_pct>"
  CAN Pack1/1 -> ETC_motorReadings1/1
  Bus Selector5/1 -> CAN Pack1/1  "<SC_motorCommand>"

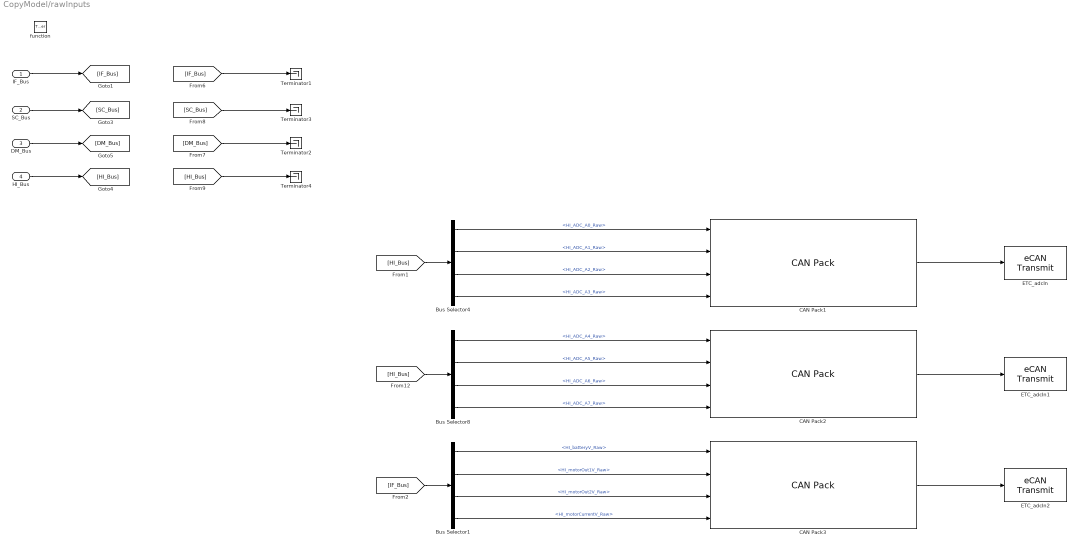
== system CopyModel/rawInputs ==
  IF_Bus : Inport
  SC_Bus : Inport  Port=2
  DM_Bus : Inport  Port=3
  HI_Bus : Inport  Port=4
  function : TriggerPort  TriggerType=function-call  VariantControl=Variant
  Bus Selector1 : BusSelector  OutputSignals=AnalogInputFiltering_Bus.OnboardADCBus.HI_batteryV_Raw,AnalogInputFiltering_Bus.OnboardADCBus.HI_motorOut1V_Raw,AnalogInputFiltering_Bus.OnboardADCBus.HI_motorOut2V_Raw,AnalogInputFiltering_Bus.OnboardADCBus.HI_motorCurrentV_Raw
  Bus Selector4 : BusSelector  OutputSignals=SPIBus.HI_ADC_A0_Raw,SPIBus.HI_ADC_A1_Raw,SPIBus.HI_ADC_A2_Raw,SPIBus.HI_ADC_A3_Raw
  Bus Selector8 : BusSelector  OutputSignals=SPIBus.HI_ADC_A4_Raw,SPIBus.HI_ADC_A5_Raw,SPIBus.HI_ADC_A6_Raw,SPIBus.HI_ADC_A7_Raw
  CAN Pack1 : canmsglib/CAN Pack  CANdbFile=C:\Git\ETC-Development\DBCs\F28377S_etc_benchTest.dbc  MsgList=ETC_adcRaw1  MsgName=ETC_adcRaw1  MsgIDType=Standard (11-bit identifier)  MsgIdentifier=1020  MsgLength=8  Remote=off  ApplyMinMax=off  BusOutput=off  SignalInfo={ 'ETC_extADC_A0_Raw', '0', '16', 'LE', 'unsigned', 'Standard', '0', '1', '0', '-Inf', 'Inf'; 'ETC_extADC_A1_Raw', '16', '16', 'LE', 'unsigned', 'Standard', '0', '1', '0', '-Inf', 'Inf'; 'ETC_extADC_A2_Raw', '32', '16', 'LE', 'unsigned', 'Standard', '0', '1', '0', '-Inf', 'Inf'; 'ETC_extADC_A3_Raw', '48', '16', 'LE', 'unsigned', 'Standard', '0', '1', '0', '-Inf', 'Inf' }
      settings: SourceProductName=Vehicle Network Toolbox  SourceProductBaseCode=VN  DataFormat=CANdb specified signals
  CAN Pack2 : canmsglib/CAN Pack  CANdbFile=C:\Git\ETC-Development\DBCs\F28377S_etc_benchTest.dbc  MsgList=ETC_adcRaw1  MsgName=ETC_adcRaw2  MsgIDType=Standard (11-bit identifier)  MsgIdentifier=1021  MsgLength=8  Remote=off  ApplyMinMax=off  BusOutput=off  SignalInfo={ 'ETC_extADC_A4_Raw', '0', '16', 'LE', 'unsigned', 'Standard', '0', '1', '0', '-Inf', 'Inf'; 'ETC_extADC_A5_Raw', '16', '16', 'LE', 'unsigned', 'Standard', '0', '1', '0', '-Inf', 'Inf'; 'ETC_extADC_A6_Raw', '32', '16', 'LE', 'unsigned', 'Standard', '0', '1', '0', '-Inf', 'Inf'; 'ETC_extADC_A7_Raw', '48', '16', 'LE', 'unsigned', 'Standard', '0', '1', '0', '-Inf', 'Inf' }
      settings: SourceProductName=Vehicle Network Toolbox  SourceProductBaseCode=VN  DataFormat=CANdb specified signals
  CAN Pack3 : canmsglib/CAN Pack  CANdbFile=C:\Git\ETC-Development\DBCs\F28377S_etc_benchTest.dbc  MsgList=ETC_adcRaw1  MsgName=ETC_adcRaw3  MsgIDType=Standard (11-bit identifier)  MsgIdentifier=1022  MsgLength=8  Remote=off  ApplyMinMax=off  BusOutput=off  SignalInfo={ 'ETC_c2000ADC_batteryVoltage_Raw', '16', '16', 'LE', 'unsigned', 'Standard', '0', '1', '0', '-Inf', 'Inf'; 'ETC_c2000ADC_motor1voltage_Raw', '32', '16', 'LE', 'unsigned', 'Standard', '0', '1', '0', '-Inf', 'Inf'; 'ETC_c2000ADC_motor2voltage_Raw', '48', '16', 'LE', 'unsigned', 'Standard', '0', '1', '0', '-Inf', 'Inf'; 'ETC_c2000ADC_motorCurrent_Raw', '0', '16', 'LE', 'unsigned', 'Standard', '0', '1', '0', '-Inf', 'Inf' }
      settings: SourceProductName=Vehicle Network Toolbox  SourceProductBaseCode=VN  DataFormat=CANdb specified signals
  ETC_adcIn : c280xlib/eCAN Transmit  chipFamily=C280x  useModule=eCAN_A  mailboxNo=5  messageID=0  messageType=Standard (11-bit identifier)  enableBlockingMode=off  postInterrupt=off  interruptLine=0
      settings: SourceProductName=Embedded Coder Support Package for Texas Instruments C2000 Processors  SourceProductBaseCode=TIC2000
  ETC_adcIn1 : c280xlib/eCAN Transmit  chipFamily=C280x  useModule=eCAN_A  mailboxNo=6  messageID=0  messageType=Standard (11-bit identifier)  enableBlockingMode=off  postInterrupt=off  interruptLine=0
      settings: SourceProductName=Embedded Coder Support Package for Texas Instruments C2000 Processors  SourceProductBaseCode=TIC2000
  ETC_adcIn2 : c280xlib/eCAN Transmit  chipFamily=C280x  useModule=eCAN_A  mailboxNo=9  messageID=0  messageType=Standard (11-bit identifier)  enableBlockingMode=off  postInterrupt=off  interruptLine=0
      settings: SourceProductName=Embedded Coder Support Package for Texas Instruments C2000 Processors  SourceProductBaseCode=TIC2000
  Terminator{1..4} (4 alike) : Terminator
  wires:
  [IF_Bus] -> Bus Selector1/1
  Bus Selector1/3 -> CAN Pack3/3  "<HI_motorOut2V_Raw>"
  CAN Pack3/1 -> ETC_adcIn2/1
  Bus Selector1/2 -> CAN Pack3/2  "<HI_motorOut1V_Raw>"
  Bus Selector1/1 -> CAN Pack3/1  "<HI_batteryV_Raw>"
  Bus Selector1/4 -> CAN Pack3/4  "<HI_motorCurrentV_Raw>"
  IF_Bus/1 -> [IF_Bus]
  [HI_Bus] -> Terminator4/1
  HI_Bus/1 -> [HI_Bus]
  SC_Bus/1 -> [SC_Bus]
  DM_Bus/1 -> [DM_Bus]
  [SC_Bus] -> Terminator3/1
  [DM_Bus] -> Terminator2/1
  [IF_Bus] -> Terminator1/1
  Bus Selector4/2 -> CAN Pack1/2  "<HI_ADC_A1_Raw>"
  Bus Selector4/3 -> CAN Pack1/3  "<HI_ADC_A2_Raw>"
  Bus Selector4/4 -> CAN Pack1/4  "<HI_ADC_A3_Raw>"
  Bus Selector8/2 -> CAN Pack2/2  "<HI_ADC_A5_Raw>"
  Bus Selector8/3 -> CAN Pack2/3  "<HI_ADC_A6_Raw>"
  Bus Selector8/4 -> CAN Pack2/4  "<HI_ADC_A7_Raw>"
  [HI_Bus] -> Bus Selector8/1
  CAN Pack2/1 -> ETC_adcIn1/1
  Bus Selector8/1 -> CAN Pack2/1  "<HI_ADC_A4_Raw>"
  CAN Pack1/1 -> ETC_adcIn/1
  [HI_Bus] -> Bus Selector4/1
  Bus Selector4/1 -> CAN Pack1/1  "<HI_ADC_A0_Raw>"

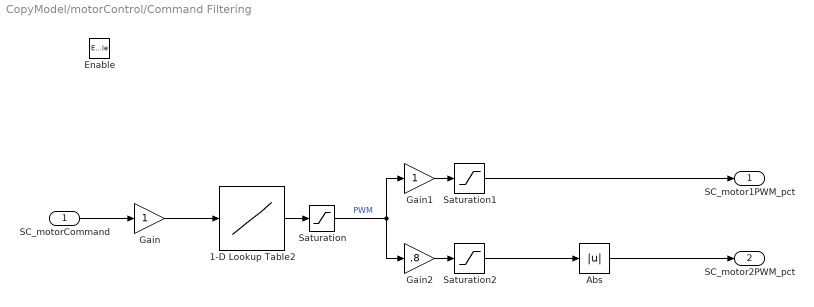
== system CopyModel/motorControl/Command Filtering ==
  SC_motorCommand : Inport
  Enable : EnablePort  StatesWhenEnabling=reset
  1-D Lookup Table2 : Lookup_n-D  NumberOfTableDimensions=1  BreakpointsForDimension1=[-100 -5 -.1 0 .1 5 100]  Table=[-100 -5 -1 0 1 20 100]  InternalRulePriority=Speed  RndMeth=Simplest  InputSameDT=on
  Abs : Abs
  Gain : Gain
  Gain1 : Gain
  Gain2 : Gain  Gain=.8
  Saturation : Saturate  UpperLimit=100  LowerLimit=-100
  Saturation1 : Saturate  UpperLimit=100  LowerLimit=0
  Saturation2 : Saturate  UpperLimit=0  LowerLimit=-100
  SC_motor1PWM_pct : Outport
  SC_motor2PWM_pct : Outport  Port=2
  wires:
  Saturation1/1 -> SC_motor1PWM_pct/1
  Saturation/1 -> Gain2/1, Gain1/1  "PWM"
  SC_motorCommand/1 -> Gain/1
  Gain2/1 -> Saturation2/1
  Gain1/1 -> Saturation1/1
  Saturation2/1 -> Abs/1
  Gain/1 -> 1-D Lookup Table2/1
  1-D Lookup Table2/1 -> Saturation/1
  Abs/1 -> SC_motor2PWM_pct/1

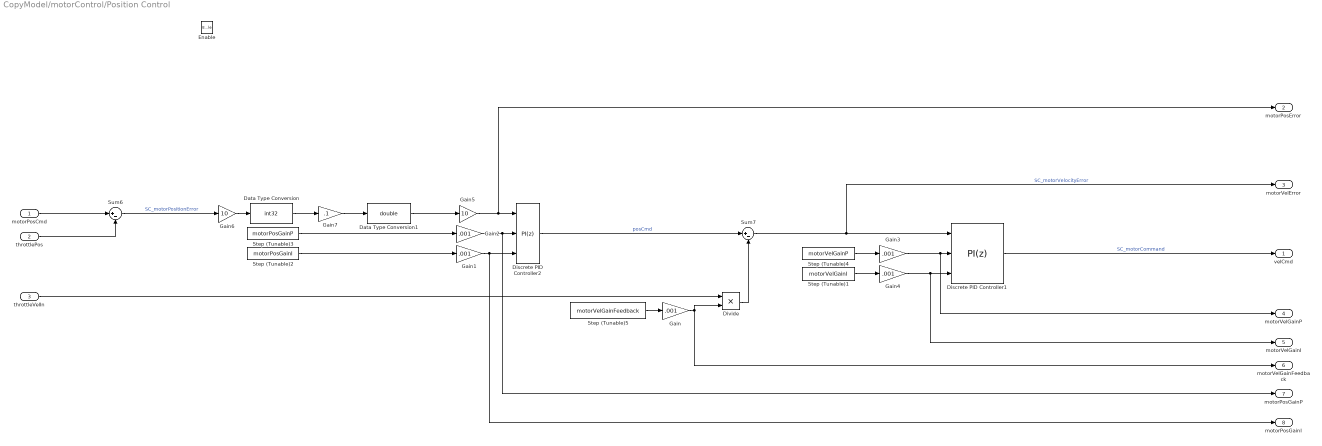
== system CopyModel/motorControl/Position Control ==
  motorPosCmd : Inport
  throttlePos : Inport  Port=2
  throttleVelIn : Inport  Port=3
  Enable : EnablePort  StatesWhenEnabling=reset
  Data Type Conversion : DataTypeConversion  OutDataTypeStr=int32
  Data Type Conversion1 : DataTypeConversion  OutDataTypeStr=double
  Discrete PID Controller1 : simulink/Continuous/PID Controller  Controller=PI  Form=Ideal  TimeDomain=Discrete-time  SampleTime=-1  IntegratorMethod=Forward Euler  FilterMethod=Forward Euler  ControllerParametersSource=external  P=0  I=0  D=0  UseFilter=off  N=100  TunerSelectOption=Transfer Function Based (PID Tuner App)  InitialConditionSource=internal  InitialConditionForIntegrator=0  InitialConditionForFilter=0  DifferentiatorICPrevScaledInput=0  ExternalReset=none  TrackingMode=off  Kt=1  LimitOutput=on  UpperSaturationLimit=100  LowerSaturationLimit=-100  LinearizeAsGain=off  AntiWindupMode=none  Kb=1  POutMin=[]  POutMax=[]  IOutMin=[]  IOutMax=[]  DOutMin=[]  DOutMax=[]  NOutMin=[]  NOutMax=[]  SumOutMin=[]  SumOutMax=[]  SaturationOutMin=[]  SaturationOutMax=[]  PParamMin=[]  PParamMax=[]  IParamMin=[]  IParamMax=[]  DParamMin=[]  DParamMax=[]  NParamMin=[]  NParamMax=[]  KbParamMin=[]  KbParamMax=[]  KtParamMin=[]  KtParamMax=[]  KbOutMin=[]  KbOutMax=[]  KtOutMin=[]  KtOutMax=[]  IntegratorOutMin=[]  IntegratorOutMax=[]  FilterOutMin=[]  FilterOutMax=[]  SumI1OutMin=[]  SumI1OutMax=[]  SumI2OutMin=[]  SumI2OutMax=[]  SumI3OutMin=[]  SumI3OutMax=[]  SumI4OutMin=[]  SumI4OutMax=[]  SumDOutMin=[]  SumDOutMax=[]  DifferentiatorOutMin=[]  DifferentiatorOutMax=[]  FilterDiffOutCoefMin=[]  FilterDiffOutCoefMax=[]  ReciprocalOutMin=[]  ReciprocalOutMax=[]  SumDenOutMin=[]  SumDenOutMax=[]  SumNumOutMin=[]  SumNumOutMax=[]  DivideOutMin=[]  DivideOutMax=[]  IntegratorContinuousStateAttributes=''  IntegratorStateMustResolveToSignalObject=off  IntegratorRTWStateStorageClass=Auto  FilterContinuousStateAttributes=''  FilterStateMustResolveToSignalObject=off  FilterRTWStateStorageClass=Auto  ParallelPVariant=Passthrough  IdealPVariant=ExternalParameters  IVariant=ExternalParameters  DVariant=Disabled  IntegratorVariant=Discrete  SatVariant=Enabled  AWVariant=Passthrough  PCopyVariant=Disabled  TRVariant=Disabled  FdbkBlocksVariant=Forward  IdealPFdbkVariant=Disabled  SatFdbkVariant=Disabled  DerivativeFilterVariant=Disabled  NVariant=Disabled  NCopyVariant=Disabled_SignalSpec  FilterICVariant=Disabled  IntegratorICVariant=InternalICs  ExternalResetVariant=Disabled  TRSumVariant=Passthrough  SumFdbkVariant=Disabled  SumVariant=Sum_PI
  Discrete PID Controller2 : simulink/Continuous/PID Controller  Controller=PI  Form=Ideal  TimeDomain=Discrete-time  SampleTime=-1  IntegratorMethod=Forward Euler  FilterMethod=Forward Euler  ControllerParametersSource=external  P=0  I=0  D=0  UseFilter=off  N=100  TunerSelectOption=Transfer Function Based (PID Tuner App)  InitialConditionSource=internal  InitialConditionForIntegrator=0  InitialConditionForFilter=0  DifferentiatorICPrevScaledInput=0  ExternalReset=none  TrackingMode=off  Kt=1  LimitOutput=on  UpperSaturationLimit=500  LowerSaturationLimit=-500  LinearizeAsGain=off  AntiWindupMode=none  Kb=1  POutMin=[]  POutMax=[]  IOutMin=[]  IOutMax=[]  DOutMin=[]  DOutMax=[]  NOutMin=[]  NOutMax=[]  SumOutMin=[]  SumOutMax=[]  SaturationOutMin=[]  SaturationOutMax=[]  PParamMin=[]  PParamMax=[]  IParamMin=[]  IParamMax=[]  DParamMin=[]  DParamMax=[]  NParamMin=[]  NParamMax=[]  KbParamMin=[]  KbParamMax=[]  KtParamMin=[]  KtParamMax=[]  KbOutMin=[]  KbOutMax=[]  KtOutMin=[]  KtOutMax=[]  IntegratorOutMin=[]  IntegratorOutMax=[]  FilterOutMin=[]  FilterOutMax=[]  SumI1OutMin=[]  SumI1OutMax=[]  SumI2OutMin=[]  SumI2OutMax=[]  SumI3OutMin=[]  SumI3OutMax=[]  SumI4OutMin=[]  SumI4OutMax=[]  SumDOutMin=[]  SumDOutMax=[]  DifferentiatorOutMin=[]  DifferentiatorOutMax=[]  FilterDiffOutCoefMin=[]  FilterDiffOutCoefMax=[]  ReciprocalOutMin=[]  ReciprocalOutMax=[]  SumDenOutMin=[]  SumDenOutMax=[]  SumNumOutMin=[]  SumNumOutMax=[]  DivideOutMin=[]  DivideOutMax=[]  IntegratorContinuousStateAttributes=''  IntegratorStateMustResolveToSignalObject=off  IntegratorRTWStateStorageClass=Auto  FilterContinuousStateAttributes=''  FilterStateMustResolveToSignalObject=off  FilterRTWStateStorageClass=Auto  ParallelPVariant=Passthrough  IdealPVariant=ExternalParameters  IVariant=ExternalParameters  DVariant=Disabled  IntegratorVariant=Discrete  SatVariant=Enabled  AWVariant=Passthrough  PCopyVariant=Disabled  TRVariant=Disabled  FdbkBlocksVariant=Forward  IdealPFdbkVariant=Disabled  SatFdbkVariant=Disabled  DerivativeFilterVariant=Disabled  NVariant=Disabled  NCopyVariant=Disabled_SignalSpec  FilterICVariant=Disabled  IntegratorICVariant=InternalICs  ExternalResetVariant=Disabled  TRSumVariant=Passthrough  SumFdbkVariant=Disabled  SumVariant=Sum_PI
  Divide : Product  Inputs=**
  Gain{,1..4} (5 alike) : Gain  Gain=.001
  Gain5 : Gain  Gain=10
  Gain6 : Gain  Gain=10
  Gain7 : Gain  Gain=.1
  Step (Tunable)1 : Constant  Value=motorVelGainI  VectorParams1D=off  SampleTime=-1
  Step (Tunable)2 : Constant  Value=motorPosGainI  VectorParams1D=off  SampleTime=-1
  Step (Tunable)3 : Constant  Value=motorPosGainP  VectorParams1D=off  SampleTime=-1
  Step (Tunable)4 : Constant  Value=motorVelGainP  VectorParams1D=off  SampleTime=-1
  Step (Tunable)5 : Constant  Value=motorVelGainFeedback  VectorParams1D=off  SampleTime=-1
  Sum6 : Sum  Inputs=|+-
  Sum7 : Sum  Inputs=|+-
  velCmd : Outport
  motorPosError : Outport  Port=2
  motorVelError : Outport  Port=3
  motorVelGainP : Outport  Port=4
  motorVelGainI : Outport  Port=5
  motorVelGainFeedback : Outport  Port=6
  motorPosGainP : Outport  Port=7
  motorPosGainI : Outport  Port=8
  wires:
  Sum6/1 -> Gain6/1  "SC_motorPositionError"
  motorPosCmd/1 -> Sum6/1
  Step (Tunable)3/1 -> Gain2/1
  Step (Tunable)2/1 -> Gain1/1
  throttlePos/1 -> Sum6/2
  Divide/1 -> Sum7/2
  Step (Tunable)1/1 -> Gain4/1
  throttleVelIn/1 -> Divide/1
  Discrete PID Controller1/1 -> velCmd/1  "SC_motorCommand"
  Sum7/1 -> Discrete PID Controller1/1, motorVelError/1  "SC_motorVelocityError"
  Step (Tunable)4/1 -> Gain3/1
  Discrete PID Controller2/1 -> Sum7/1  "posCmd"
  Step (Tunable)5/1 -> Gain/1
  Gain/1 -> motorVelGainFeedback/1, Divide/2
  Gain1/1 -> motorPosGainI/1, Discrete PID Controller2/3
  Gain2/1 -> motorPosGainP/1, Discrete PID Controller2/2
  Gain3/1 -> motorVelGainP/1, Discrete PID Controller1/2
  Gain4/1 -> motorVelGainI/1, Discrete PID Controller1/3
  Gain5/1 -> motorPosError/1, Discrete PID Controller2/1
  Gain6/1 -> Data Type Conversion/1
  Gain7/1 -> Data Type Conversion1/1
  Data Type Conversion/1 -> Gain7/1
  Data Type Conversion1/1 -> Gain5/1
